simulink model "R_S_P_block"  (R2021a)
settings: Solver=VariableStepAuto  StartTime=0.0  StopTime=10.0  RelTol=1e-3
settings Model: Creator=Nabil  LastModifiedBy=Nabil

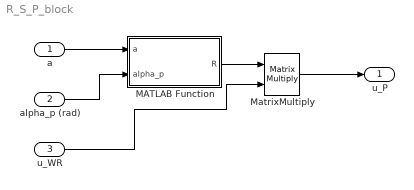
== system R_S_P_block ==
  a : Inport
  alpha_p (rad) : Inport  Port=2
  u_WR : Inport  Port=3  PortDimensions=3
  MATLAB Function : MATLAB Function  TreatAsAtomicUnit=on
  MatrixMultiply : Product  Multiplication=Matrix(*)
  u_P : Outport
  wires:
  u_WR/1 -> MatrixMultiply/2
  MatrixMultiply/1 -> u_P/1
  a/1 -> MATLAB Function/1(a)
  alpha_p (rad)/1 -> MATLAB Function/2(alpha_p)
  MATLAB Function/1(R) -> MatrixMultiply/1

== matlab function R_S_P_block/MATLAB Function ==
  data: a input; R output; alpha_p input
function R = fcn(a, alpha_p)

R = R_S_P(a, alpha_p);
